simulink model "MPC_emulator"  (R2025a)
settings: Solver=VariableStepAuto  StartTime=0.0  StopTime=10  RelTol=1e-3
values from neighbouring files (symbols this model uses):
  a = .15    (= 0.15)    [UGV_Discrete_Time_Dynamics.m]
  b = .15    (= 0.15)    [UGV_Discrete_Time_Dynamics.m]
  Cf = 70    [UGV_Discrete_Time_Dynamics.m]
  Iz = .05    (= 0.05)    [UGV_Discrete_Time_Dynamics.m]
  m = 5    [UGV_Discrete_Time_Dynamics.m]
  Pvx = 10    [UGV_Discrete_Time_Dynamics.m]
libraries: vehdynlibdriver x1, slpidlib x1, simulink x1, SignalEditorBlockLib x1
settings Model: Creator=bshla  LastModifiedBy=bshla

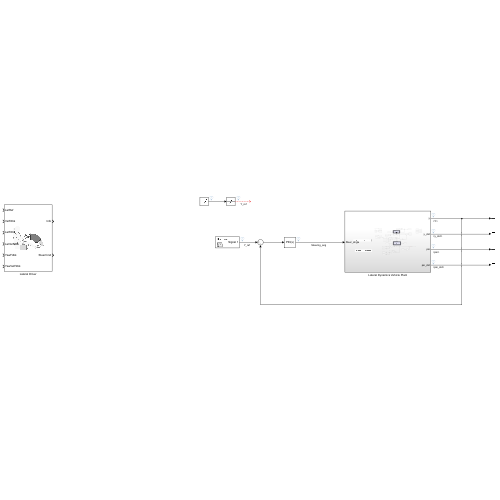
[thumbnail: Simulink's stored preview of the top-level diagram]
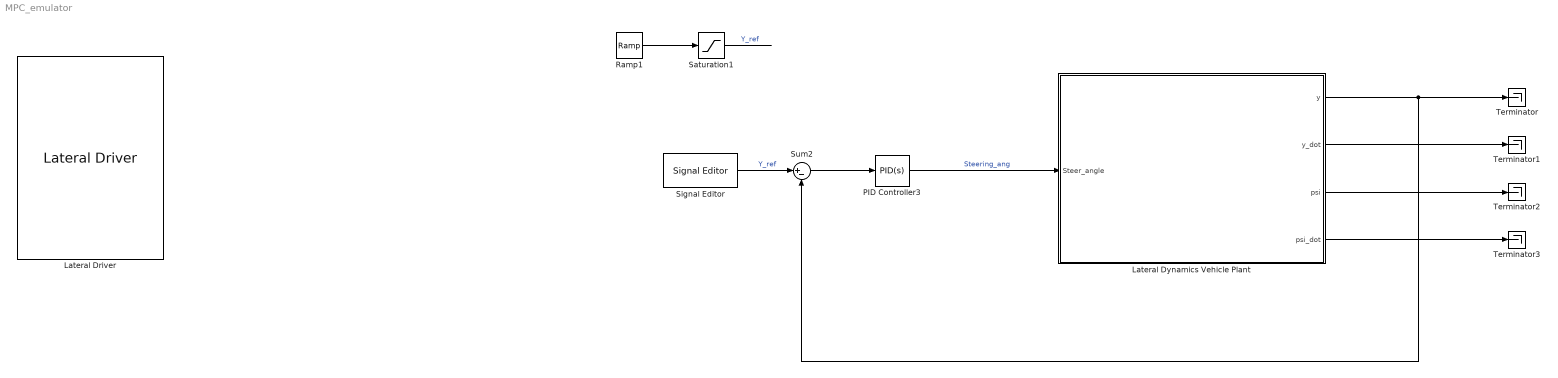
== system MPC_emulator ==
  Lateral Driver : vehdynlibdriver/Lateral Driver  extSteerOvr=off  extSteerHld=off  extSteerZero=off  steerOut=off  cntrlTypeLat=Predictive  coordMode=SAE J670 (Z-down)  angUnits=rad  tau=0.1  L=3  vecPose=off  dynamMode=off  PositionGainF=2.5  PositionGainR=2.5  YawRateGain=.2  DelayGain=.2  a=1.41  b=1.41  m=2016  Cy_f=25266  Cy_r=70933  I=4013  Ksteer=18  theta=45*pi/180  aMode=2
  Lateral Dynamics Vehicle Plant : Subsystem
  PID Controller3 : slpidlib/PID Controller  Controller=PID  Form=Parallel  TimeDomain=Continuous-time  UseExternalTs=off  SampleTime=-1  IntegratorMethod=Forward Euler  FilterMethod=Forward Euler  ControllerParametersSource=internal  P=5  I=0  UseKiTs=off  D=2  UseExternalDerivativeSource=off  N=100  UseFilter=on  TunerSelectOption=Transfer Function Based (PID Tuner App)  InitialConditionSource=internal  InitialConditionForIntegrator=0  InitialConditionForFilter=0  DifferentiatorICPrevScaledInput=0  ExternalReset=none  TrackingMode=off  Kt=1  LimitOutput=off  SatLimitsSource=internal  UpperSaturationLimit=inf  LowerSaturationLimit=-inf  LinearizeAsGain=on  AntiWindupMode=none  Kb=1  LimitIntegrator=off  UpperIntegratorSaturationLimit=inf  LowerIntegratorSaturationLimit=-inf  POutMin=[]  POutMax=[]  IOutMin=[]  IOutMax=[]  DOutMin=[]  DOutMax=[]  NOutMin=[]  NOutMax=[]  SumOutMin=[]  SumOutMax=[]  SaturationOutMin=[]  SaturationOutMax=[]  PParamMin=[]  PParamMax=[]  IParamMin=[]  IParamMax=[]  DParamMin=[]  DParamMax=[]  NParamMin=[]  NParamMax=[]  KbParamMin=[]  KbParamMax=[]  KtParamMin=[]  KtParamMax=[]  KbOutMin=[]  KbOutMax=[]  KtOutMin=[]  KtOutMax=[]  IntegratorOutMin=[]  IntegratorOutMax=[]  FilterOutMin=[]  FilterOutMax=[]  SumI1OutMin=[]  SumI1OutMax=[]  SumI2OutMin=[]  SumI2OutMax=[]  SumI3OutMin=[]  SumI3OutMax=[]  SumI4OutMin=[]  SumI4OutMax=[]  SumDOutMin=[]  SumDOutMax=[]  DifferentiatorOutMin=[]  DifferentiatorOutMax=[]  FilterDiffOutCoefMin=[]  FilterDiffOutCoefMax=[]  ReciprocalOutMin=[]  ReciprocalOutMax=[]  SumDenOutMin=[]  SumDenOutMax=[]  SumNumOutMin=[]  SumNumOutMax=[]  DivideOutMin=[]  DivideOutMax=[]  UdiffTsProdOutMin=[]  UdiffTsProdOutMax=[]  NTsProdOutMin=[]  NTsProdOutMax=[]  UintegralTsProdOutMin=[]  UintegralTsProdOutMax=[]  UngainTsProdOutMin=[]  UngainTsProdOutMax=[]  ClampingZeroOutDataTypeStr=Inherit: Inherit via back propagation  ClampingZeroOutMin=[]  ClampingZeroOutMax=[]  FilterDenConstantOutDataTypeStr=Inherit: Inherit via back propagation  FilterDenConstantOutMin=[]  FilterDenConstantOutMax=[]  PCopyOutDataTypeStr=Inherit: Inherit via back propagation  PCopyOutMin=[]  PCopyOutMax=[]  NCopyOutDataTypeStr=Inherit: Inherit via back propagation  NCopyOutMin=[]  NCopyOutMax=[]  IntegratorContinuousStateAttributes=''  IntegratorStateMustResolveToSignalObject=off  IntegratorRTWStateStorageClass=Auto  FilterContinuousStateAttributes=''  FilterStateMustResolveToSignalObject=off  FilterRTWStateStorageClass=Auto  ParallelPVariant=InternalParameters  IdealPVariant=Disabled  IVariant=InternalParameters  DVariant=InternalParameters  IntegratorVariant=Continuous  SatVariant=Disabled  AWVariant=Passthrough  PCopyVariant=Disabled  TRVariant=Disabled  FdbkBlocksVariant=Forward  IdealPFdbkVariant=Disabled  SatFdbkVariant=Disabled  DerivativeFilterVariant=ContFilter  NVariant=InternalParameters  NCopyVariant=Disabled  FilterICVariant=InternalICsFilter  IntegratorICVariant=InternalICs  ExternalResetVariant=Disabled  TRSumVariant=Passthrough  SumFdbkVariant=Disabled  SumVariant=Sum_PID  TsampFilterVariant=InternalTs  TsampNgainVariant=Passthrough  TsampIntegralVariant=Disabled_SignalSpec  ExternalSaturationOutDataTypeStr=Inherit: Same as second input  DerivativeSourceVariant=ErrorSignal  PreIntVariant=InternalPreInt
  Ramp1 : simulink/Sources/Ramp  slope=0.25  start=0  InitialOutput=0
  Saturation1 : Saturate  UpperLimit=1  LowerLimit=-1
  Signal Editor : SignalEditorBlockLib/Signal Editor  FileName=lane change.mat  ActiveScenario=Scenario  ActiveSignal=Signal 1  IsBus=off  OutputBusObjectStr=Bus: BusObject  SampleTime=0  ZeroCross=off  OutputAfterFinalValue=Setting to zero  Unit=inherit  PreserveSignalName=on  ApplySigPropsToAllScenarios=on  ApplySigPropsToAllSignals=off  SignalPropertySource=Dialog parameters
  Sum2 : Sum  Inputs=|+-
  Terminator{,1..3} (4 alike) : Terminator
  wires:
  Lateral Dynamics Vehicle Plant/1(y) -> Sum2/2, Terminator/1
  Lateral Dynamics Vehicle Plant/2(y_dot) -> Terminator1/1
  Lateral Dynamics Vehicle Plant/3(psi) -> Terminator2/1
  Lateral Dynamics Vehicle Plant/4(psi_dot) -> Terminator3/1
  Signal Editor/1 -> Sum2/1  "Y_ref"
  PID Controller3/1 -> Lateral Dynamics Vehicle Plant/1(Steer_angle)  "Steering_ang"
  Sum2/1 -> PID Controller3/1
  Ramp1/1 -> Saturation1/1
  Saturation1/1 -> ?  "Y_ref"

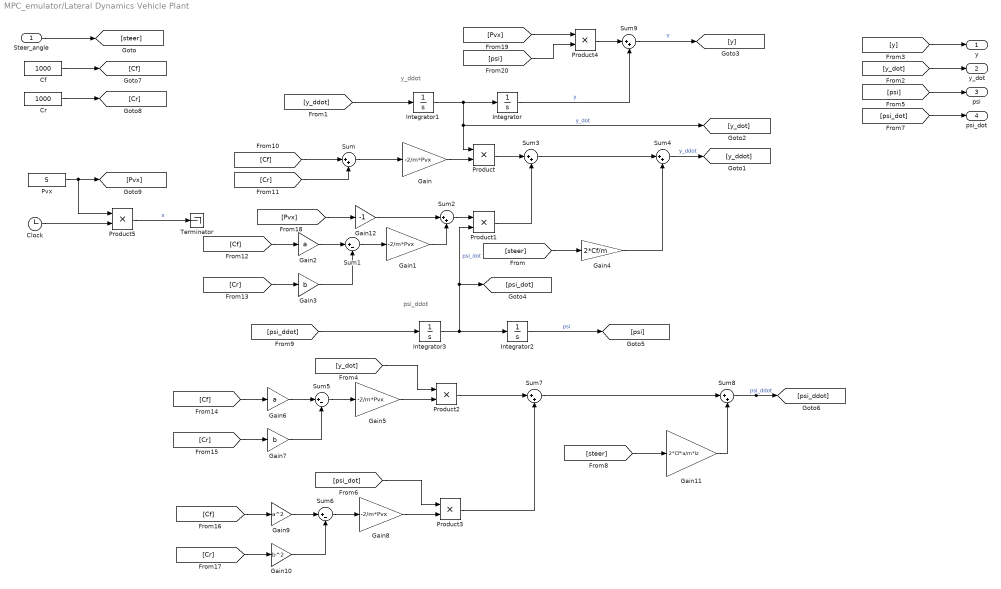
== system MPC_emulator/Lateral Dynamics Vehicle Plant ==
  note: psi_ddot
  note: y_ddot
  Steer_angle : Inport
  Cf : Constant  Value=1000
  Clock : Clock
  Cr : Constant  Value=1000
  Gain{,1,5,8} (4 alike) : Gain  Gain=-2/m*Pvx
  Gain10 : Gain  Gain=b^2
  Gain11 : Gain  Gain=2*Cf*a/m*Iz
  Gain12 : Gain  Gain=-1
  Gain2 : Gain  Gain=a
  Gain3 : Gain  Gain=b
  Gain4 : Gain  Gain=2*Cf/m
  Gain6 : Gain  Gain=a
  Gain7 : Gain  Gain=b
  Gain9 : Gain  Gain=a^2
  Integrator{,1..3} (4 alike) : Integrator
  Product{,1..5} (6 alike) : Product
  Pvx : Constant  Value=5
  Sum{,2..4,7..9} (7 alike) : Sum  Inputs=|++
  Sum1 : Sum  Inputs=|+-
  Sum5 : Sum  Inputs=|+-
  Sum6 : Sum  Inputs=|+-
  Terminator : Terminator
  y : Outport
  y_dot : Outport  Port=2
  psi : Outport  Port=3
  psi_dot : Outport  Port=4
  wires:
  Integrator1/1 -> Product/1, [y_dot], Integrator/1  "y_dot"
  Sum/1 -> Gain/1
  Sum1/1 -> Gain1/1
  [Cr] -> Gain3/1
  [Cf] -> Gain2/1
  Gain2/1 -> Sum1/1
  Gain3/1 -> Sum1/2
  Gain1/1 -> Sum2/2
  Gain/1 -> Product/2
  Product/1 -> Sum3/1
  Sum2/1 -> Product1/1
  Product1/1 -> Sum3/2
  Steer_angle/1 -> [steer]
  [steer] -> Gain4/1
  Gain4/1 -> Sum4/2
  Sum3/1 -> Sum4/1
  Sum5/1 -> Gain5/1
  Gain5/1 -> Product2/2
  Gain6/1 -> Sum5/1
  [Cf] -> Gain6/1
  Gain7/1 -> Sum5/2
  [Cr] -> Gain7/1
  Sum4/1 -> [y_ddot]  "y_ddot"
  [y_ddot] -> Integrator1/1
  [y_dot] -> y_dot/1
  [y] -> y/1
  Product2/1 -> Sum7/1
  [y_dot] -> Product2/1
  [psi_dot] -> Product3/1
  Product3/1 -> Sum7/2
  [Cr] -> Gain10/1
  Gain10/1 -> Sum6/2
  [Cf] -> Gain9/1
  Gain9/1 -> Sum6/1
  Gain8/1 -> Product3/2
  Sum6/1 -> Gain8/1
  Integrator3/1 -> Integrator2/1, [psi_dot], Product1/2  "psi_dot"
  Integrator2/1 -> [psi]  "psi"
  [psi] -> psi/1
  [psi_dot] -> psi_dot/1
  [steer] -> Gain11/1
  Sum7/1 -> Sum8/1
  Gain11/1 -> Sum8/2
  Sum8/1 -> [psi_ddot]  "psi_ddot"
  [psi_ddot] -> Integrator3/1
  Cf/1 -> [Cf]
  Cr/1 -> [Cr]
  [Cf] -> Sum/1
  [Cr] -> Sum/2
  Sum9/1 -> [y]  "Y"
  Pvx/1 -> Product5/1, [Pvx]
  [Pvx] -> Gain12/1
  Product4/1 -> Sum9/1
  [Pvx] -> Product4/1
  [psi] -> Product4/2
  Integrator/1 -> Sum9/2  "y"
  Gain12/1 -> Sum2/1
  Clock/1 -> Product5/2
  Product5/1 -> Terminator/1  "x"
